simulink model "OT_model"  (R2022b)
settings: Solver=VariableStepAuto  StartTime=0.0  StopTime=10.0  RelTol=1e-3
values from neighbouring files (symbols this model uses):
  air_den = 1.225    [wind_turbine_parameters.m]
  B = 10    [wind_turbine_parameters.m]
  J = 100    [wind_turbine_parameters.m]
  K_op = 0.5*air_den*pi*power(l1,5)*Cp_max/power(lambda_op,3)    [wind_turbine_parameters.m]
  l1 = 56    [wind_turbine_parameters.m]
  t_sample = 10*60    (= 600)    [wind_turbine_parameters.m]
libraries: spsWindTurbineLib x1
settings Model: Creator=marina  LastModifiedBy=marina

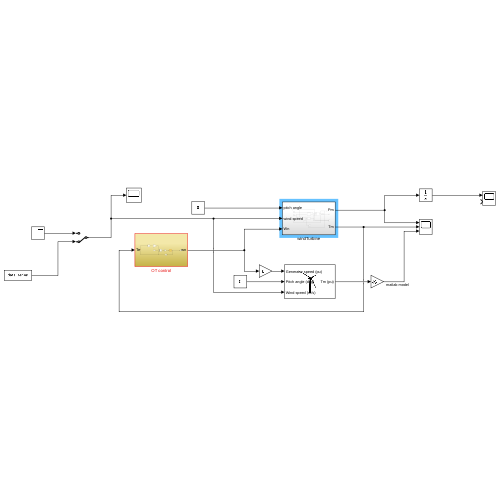
[thumbnail: Simulink's stored preview of the top-level diagram]
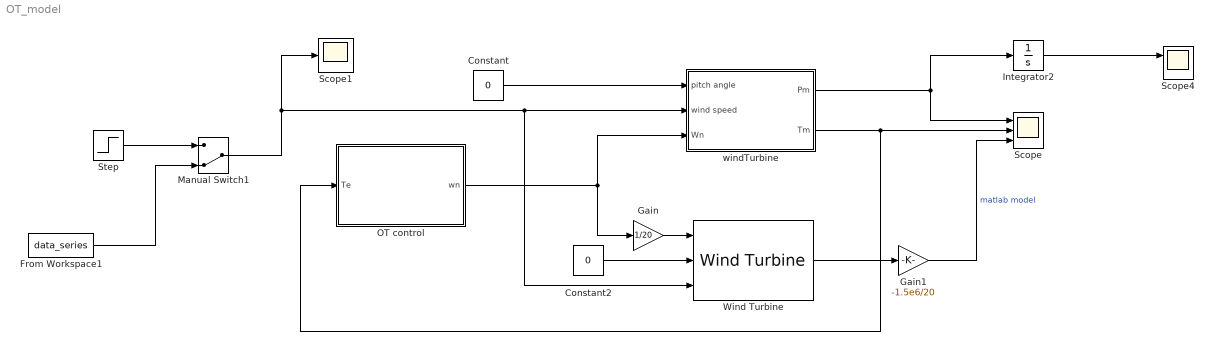
== system OT_model ==
  Constant : Constant  Value=0
  Constant2 : Constant  Value=0
  From Workspace1 : FromWorkspace  VariableName=data_series  SampleTime=t_sample  OutputAfterFinalValue=Holding final value
  Gain : Gain  Gain=1/20
  Gain1 : Gain  Gain=-1.5e6/20
  Integrator2 : Integrator
  Manual Switch1 : ManualSwitch  CurrentSetting=0
  OT control : Subsystem
  Scope : Scope  NumInputPorts=3
  Scope1 : Scope
  Scope4 : Scope  NumInputPorts=2
  Step : Step  Time=0  Before=1  After=20  SampleTime=0
  Wind Turbine : spsWindTurbineLib/Wind Turbine  Pnom=1.5e6  Pelec_base=1.5e6/0.9  wind_base=4  P_wind_base=0.73  speed_nom=1.2  pitch_angle=0  c1_c6="[0.51763          116          0.4            5           21     0.006795]"  cp_nom=0.48  lambda_nom=8.1
  windTurbine : Subsystem
  wires:
  From Workspace1/1 -> Manual Switch1/2
  Integrator2/1 -> Scope4/1
  Manual Switch1/1 -> Wind Turbine/3, windTurbine/2(wind speed), Scope1/1
  Constant2/1 -> Wind Turbine/2
  Wind Turbine/1 -> Gain1/1
  Step/1 -> Manual Switch1/1
  OT control/1(wn) -> windTurbine/3(Wn), Gain/1
  windTurbine/2(Tm) -> OT control/1(Te), Scope/2
  Constant/1 -> windTurbine/1(pitch angle)
  windTurbine/1(Pm) -> Integrator2/1, Scope/1
  Gain/1 -> Wind Turbine/1
  Gain1/1 -> Scope/3  "matlab model"

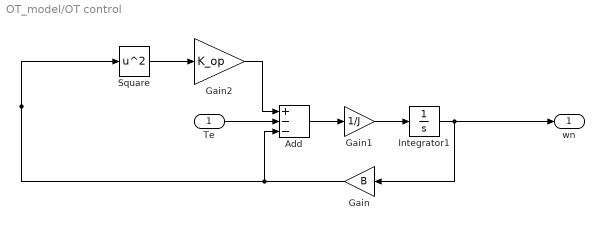
== system OT_model/OT control ==
  Te : Inport
  Add : Sum  Inputs=+--
  Gain : Gain  Gain=B
  Gain1 : Gain  Gain=1/J
  Gain2 : Gain  Gain=K_op
  Integrator1 : Integrator  InitialCondition=0.000001
  Square : Math  Operator=square
  wn : Outport
  wires:
  Te/1 -> Add/2
  Gain1/1 -> Integrator1/1
  Add/1 -> Gain1/1
  Square/1 -> Gain2/1
  Integrator1/1 -> Gain/1, wn/1
  Gain/1 -> Square/1, Add/3
  Gain2/1 -> Add/1

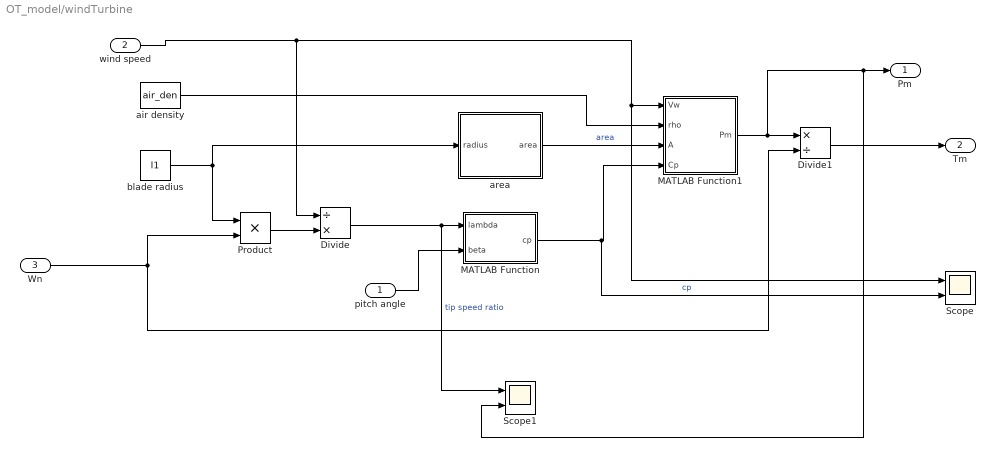
== system OT_model/windTurbine ==
  pitch angle : Inport
  wind speed : Inport  Port=2
  Wn : Inport  Port=3
  Divide : Product  Inputs=/*
  Divide1 : Product  Inputs=*/
  MATLAB Function : MATLAB Function  TreatAsAtomicUnit=on
  MATLAB Function1 : MATLAB Function  TreatAsAtomicUnit=on
  Product : Product
  Scope : Scope  NumInputPorts=2
  Scope1 : Scope  NumInputPorts=2
  air density : Constant  Value=air_den
  area : Subsystem
  blade radius : Constant  Value=l1
  Pm : Outport
  Tm : Outport  Port=2
  wires:
  blade radius/1 -> Product/1, area/1(radius)
  Product/1 -> Divide/2
  wind speed/1 -> Scope/1, MATLAB Function1/1(Vw), Divide/1
  Divide/1 -> Scope1/1, MATLAB Function/1(lambda)  "tip speed ratio"
  pitch angle/1 -> MATLAB Function/2(beta)
  area/1(area) -> MATLAB Function1/3(A)  "area"
  MATLAB Function/1(cp) -> Scope/2, MATLAB Function1/4(Cp)  "cp"
  MATLAB Function1/1(Pm) -> Divide1/1, Scope1/2, Pm/1
  Divide1/1 -> Tm/1
  air density/1 -> MATLAB Function1/2(rho)
  Wn/1 -> Divide1/2, Product/2

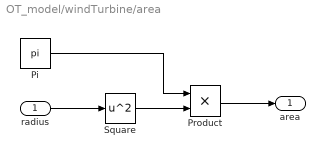
== system OT_model/windTurbine/area ==
  radius : Inport
  Pi : Constant  Value=pi  OutDataTypeStr=Inherit: Inherit via back propagation
  Product : Product
  Square : Math  Operator=square
  area : Outport
  wires:
  radius/1 -> Square/1
  Square/1 -> Product/2
  Pi/1 -> Product/1
  Product/1 -> area/1

== matlab function OT_model/windTurbine/MATLAB Function1 ==
  data: Vw input; Pm output; rho input; A input; Cp input
function Pm = fcn(Vw, rho, A, Cp)

Pm = 0.5* Cp* rho* A* power(Vw, 3);

== matlab function OT_model/windTurbine/MATLAB Function ==
  data: lambda input; cp output; beta input
function cp = fcn(lambda, beta)

k = load('coefficients.mat');
lambda_i =  1/(1/(lambda + 0.08*beta) - 0.035/(1+beta*beta*beta));

% Debug
% lambda_i
% k.k1 *(k.k2/lambda_i - k.k3*beta - k.k4*power(beta, k.k5) -k.k6)*exp(-k.k7/lambda_i)

cp = k.k1 *(k.k2/lambda_i - k.k3*beta - k.k4*power(beta, k.k5) -k.k6)*exp(-k.k7/lambda_i);
